simulink model "PROJE_Bolum1"  (R2018b)
settings: Solver=VariableStepAuto  StartTime=0.0  StopTime=20  RelTol=1e-3
InitFcn:
  | m1=300;
  | m2=200;
  | m3=100;
  | m4=300;
  | m5=500;
  | k1=500;
  | k2=200;
  | k3=100;
  | k4=400;
  | k5=500;
  | k6=600;
  | a1=300;
  | a2=450;
  | a3=300;
  | a4=400;
  | a5=500;
  | a6=600;
  | c1=300;
  | c2=200;
  | c3=100;
  | c4=400;
  | c5=550;
  | c6=250;
  | delta1=200;
  | delta2=500;
  | delta3=400;
  | delta4=300;
  | delta5=100;
  | omega1=30;
  | omega2=50;
  | omega3=80;
  | omega4=20;
  | omega5=100;
settings Model: Creator=Fatih  LastModifiedBy=Fatih

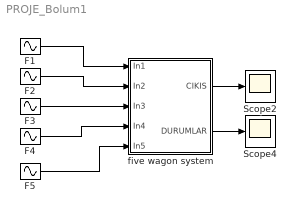
== system PROJE_Bolum1 ==
  F1 : Sin  Amplitude=delta1  Frequency=omega1  SampleTime=0
  F2 : Sin  Amplitude=delta2  Frequency=omega2  SampleTime=0
  F3 : Sin  Amplitude=delta3  Frequency=omega3  SampleTime=0
  F4 : Sin  Amplitude=delta4  Frequency=omega4  SampleTime=0
  F5 : Sin  Amplitude=delta5  Frequency=omega5  SampleTime=0
  Scope2 : Scope
  Scope4 : Scope
  "five wagon system " : Subsystem
  wires:
  F5/1 -> "five wagon system "/5(In5)
  F2/1 -> "five wagon system "/2(In2)
  F4/1 -> "five wagon system "/4(In4)
  "five wagon system "/1(CIKIS) -> Scope2/1
  F1/1 -> "five wagon system "/1(In1)
  F3/1 -> "five wagon system "/3(In3)
  "five wagon system "/2("DURUMLAR ") -> Scope4/1

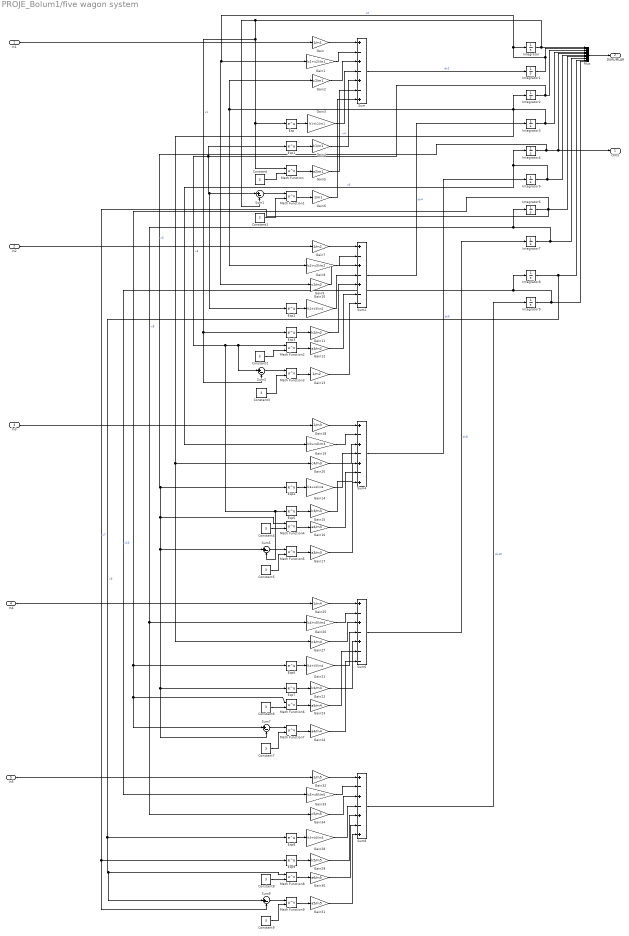
== system PROJE_Bolum1/five wagon system  ==
  In1 : Inport
  In2 : Inport  Port=2
  In3 : Inport  Port=3
  In4 : Inport  Port=4
  In5 : Inport  Port=5
  Constant{,1..9} (10 alike) : Constant  Value=3
  Exp{,1..9} (10 alike) : Math  SaturateOnIntegerOverflow=on
  Gain : Gain  Gain=1/m1
  Gain1 : Gain  Gain=(c1+c2)/m1
  Gain10 : Gain  Gain=(k2+k3)/m2
  Gain11 : Gain  Gain=k2/m2
  Gain12 : Gain  Gain=a3/m2
  Gain13 : Gain  Gain=1/m2
  Gain14 : Gain  Gain=(k3+k4)/m3
  Gain15 : Gain  Gain=k3/m3
  Gain16 : Gain  Gain=a4/m3
  Gain17 : Gain  Gain=a3/m3
  Gain18 : Gain  Gain=1/m3
  Gain19 : Gain  Gain=(c3+c4)/m3
  Gain2 : Gain  Gain=c2/m1
  Gain20 : Gain  Gain=c4/m3
  Gain21 : Gain  Gain=(k4+k5)/m4
  Gain22 : Gain  Gain=k4/m4
  Gain23 : Gain  Gain=a5/m4
  Gain24 : Gain  Gain=a4/m4
  Gain25 : Gain  Gain=1/m4
  Gain26 : Gain  Gain=(c4+c5)/m4
  Gain27 : Gain  Gain=c4/m4
  Gain28 : Gain  Gain=(k5+k6)/m5
  Gain29 : Gain  Gain=k5/m5
  Gain3 : Gain  Gain=(k1+k2)/m1
  Gain30 : Gain  Gain=a6/m5
  Gain31 : Gain  Gain=a5/m5
  Gain32 : Gain  Gain=1/m5
  Gain33 : Gain  Gain=(c5+c6)/m5
  Gain34 : Gain  Gain=c5/m5
  Gain4 : Gain  Gain=k1/m1
  Gain5 : Gain  Gain=a2/m1
  Gain6 : Gain  Gain=1/m1
  Gain7 : Gain  Gain=1/m2
  Gain8 : Gain  Gain=(c2+c3)/m2
  Gain9 : Gain  Gain=c2/m2
  Integrator{,1..9} (10 alike) : Integrator
  Math Function{,1..9} (10 alike) : Math  Operator=pow  SaturateOnIntegerOverflow=on
  Mux : Mux  Inputs=10
  Sum : Sum  Inputs=+-+-+-+
  Sum{1,3,5,7,9} (5 alike) : Sum  Inputs=|+-
  Sum2 : Sum  Inputs=+-+-+--
  Sum4 : Sum  Inputs=+-+-+-+
  Sum6 : Sum  Inputs=+-+-+--
  Sum8 : Sum  Inputs=+-+-+-+
  CIKIS : Outport
  "DURUMLAR " : Outport  Port=2
  wires:
  Gain19/1 -> Sum4/2
  Constant9/1 -> Math Function9/2
  Constant8/1 -> Math Function8/2
  Exp6/1 -> Gain21/1
  Exp5/1 -> Gain15/1
  Exp9/1 -> Gain29/1
  Gain30/1 -> Sum8/6
  In2/1 -> Gain7/1
  Gain22/1 -> Sum6/5
  Math Function5/1 -> Gain17/1
  Gain20/1 -> Sum4/3
  Exp7/1 -> Gain22/1
  Gain25/1 -> Sum6/1
  Gain32/1 -> Sum8/1
  Sum5/1 -> Math Function5/1
  Constant4/1 -> Math Function4/2
  Exp4/1 -> Gain14/1
  Constant2/1 -> Math Function2/2
  Gain14/1 -> Sum4/4
  Gain16/1 -> Sum4/6
  Gain15/1 -> Sum4/5
  Gain13/1 -> Sum2/7
  Sum4/1 -> Integrator5/1  "dx6"
  Gain6/1 -> Sum/7
  Math Function1/1 -> Gain6/1
  Math Function8/1 -> Gain30/1
  Exp2/1 -> Gain10/1
  Sum9/1 -> Math Function9/1
  Gain3/1 -> Sum/4
  Sum1/1 -> Math Function1/1
  Sum8/1 -> Integrator9/1  "dx10"
  Gain24/1 -> Sum6/7
  Math Function2/1 -> Gain12/1
  In4/1 -> Gain25/1
  Constant6/1 -> Math Function6/2
  In1/1 -> Gain/1
  Gain31/1 -> Sum8/7
  Mux/1 -> "DURUMLAR "/1
  Constant/1 -> Math Function/2
  Gain2/1 -> Sum/3
  Gain/1 -> Sum/1
  Constant7/1 -> Math Function7/2
  Math Function4/1 -> Gain16/1
  Sum3/1 -> Math Function3/1
  Sum7/1 -> Math Function7/1
  Exp1/1 -> Gain4/1
  Math Function3/1 -> Gain13/1
  Math Function6/1 -> Gain23/1
  Gain17/1 -> Sum4/7
  In5/1 -> Gain32/1
  Sum2/1 -> Integrator3/1  "dx4"
  Gain33/1 -> Sum8/2
  Integrator9/1 -> Gain33/1, Integrator8/1, Mux/10  "x10"
  Gain23/1 -> Sum6/6
  Constant5/1 -> Math Function5/2
  Gain28/1 -> Sum8/4
  In3/1 -> Gain18/1
  Integrator1/1 -> Mux/2, Gain9/1, Gain1/1, Integrator/1  "x2"
  Gain5/1 -> Sum/6
  Gain8/1 -> Sum2/2
  Gain27/1 -> Sum6/3
  Sum/1 -> Integrator1/1  "dx2"
  Sum6/1 -> Integrator7/1  "dx8"
  Gain11/1 -> Sum2/5
  Integrator7/1 -> Gain34/1, Gain26/1, Integrator6/1, Mux/8  "x8"
  Gain7/1 -> Sum2/1
  Integrator3/1 -> Integrator2/1, Gain2/1, Gain8/1, Gain27/1, Gain20/1, Mux/4  "x4"
  Gain21/1 -> Sum6/4
  Gain1/1 -> Sum/2
  Constant1/1 -> Math Function1/2
  Integrator5/1 -> Gain19/1, Integrator4/1, Mux/6  "x6"
  Gain29/1 -> Sum8/5
  Exp3/1 -> Gain11/1
  Exp/1 -> Gain3/1
  Math Function7/1 -> Gain24/1
  Gain12/1 -> Sum2/6
  Gain26/1 -> Sum6/2
  Integrator2/1 -> Mux/3, Sum5/2, Exp5/1, Sum3/1, Math Function2/1, Sum1/1, Exp2/1, Exp1/1  "x3"
  Gain9/1 -> Sum2/3
  Integrator4/1 -> Sum7/2, Exp7/1, Sum5/1, Math Function4/1, Exp4/1, CIKIS/1, Mux/5  "x5"
  Exp8/1 -> Gain28/1
  Gain4/1 -> Sum/5
  Integrator8/1 -> Sum9/1, Math Function8/1, Exp8/1, Mux/9  "x9"
  Math Function/1 -> Gain5/1
  Gain18/1 -> Sum4/1
  Gain34/1 -> Sum8/3
  Math Function9/1 -> Gain31/1
  Integrator/1 -> Exp/1, Math Function/1, Exp3/1, Sum3/2, Sum1/2, Mux/1  "x1"
  Integrator6/1 -> Sum9/2, Exp9/1, Sum7/1, Math Function6/1, Exp6/1, Mux/7  "x7"
  Constant3/1 -> Math Function3/2
  Gain10/1 -> Sum2/4
